simulink model "LIVA_AUV_SIMULATOR"  (R2023b)
settings: Solver=ode4  StartTime=0.0  StopTime=100  FixedStep=0.001  RelTol=0.01  EnableMultiTasking=on
InitFcn:
  | LIVA_AUV_Simulator_init;
model workspace (MAT data in the model file):
  a = 0.0768559116543
  a1 = 5.09287831845
  b = 2.78447714902
  b1 = 0.0150573456987
  c = 0.222680447107
  c1 = 0.0244981849866
  d = 1.17025942432
  d1 = -0.121090969634
  e = 4
  e1 = -0.000744741765672
  f = 3.22045295126
  f1 = 0.147531958158
  g = 3
  g1 = 9.31921319068e-05
  h = 4
  h1 = -0.000787888183232
  i = 2.39426372075
  i1 = -0.0976897881188
  j = 3
  j1 = 7.29765081481
  k = 2
  k1 = 3.34164431501
  l = -0.0819081975806
  l1 = 4.85550524224
  m = -0.0907196254339
  m1 = 2.91684244028
  n = 1.20537954163
  n1 = 9.00648148706
  o = 1.92822193114
  o1 = 2.79427167815
  p = 1.9547800679
  p1 = 9.64465760947
  r = 2
  r1 = 9.85880905818
  s = 0.00182097897058
  s1 = 6.72892013716
values from neighbouring files (symbols this model uses):
  alfa = 1.1    [LIVA_AUV_Simulator_init.m]
  B = 114.8*pk    (= 149.24)    [LIVA_AUV_Simulator_init.m]
  Hybrid_pKd = 1.9282219311449538    (= 1.92822193114)    [LIVA_AUV_Simulator_init.m]
  Hybrid_pKi = 1.205379541632126    (= 1.20537954163)    [LIVA_AUV_Simulator_init.m]
  Hybrid_pKp = -0.090719625433908213    (= -0.0907196254339)    [LIVA_AUV_Simulator_init.m]
  Hybrid_rKd = -0.0819081975805605    (= -0.0819081975806)    [LIVA_AUV_Simulator_init.m]
  Hybrid_rKi = 2    [LIVA_AUV_Simulator_init.m]
  Hybrid_rKp = 3    [LIVA_AUV_Simulator_init.m]
  Hybrid_xalfa = 5.092878318451735    (= 5.09287831845)    [LIVA_AUV_Simulator_init.m]
  Hybrid_xbeta = 0.024498184986623803    (= 0.0244981849866)    [LIVA_AUV_Simulator_init.m]
  Hybrid_xKd = 0.22268044710682114    (= 0.222680447107)    [LIVA_AUV_Simulator_init.m]
  Hybrid_xKi = 2.7844771490230995    (= 2.78447714902)    [LIVA_AUV_Simulator_init.m]
  Hybrid_xKp = 0.076855911654313547    (= 0.0768559116543)    [LIVA_AUV_Simulator_init.m]
  Hybrid_yalfa = -0.12109096963388193    (= -0.121090969634)    [LIVA_AUV_Simulator_init.m]
  Hybrid_ybeta = 0.14753195815811565    (= 0.147531958158)    [LIVA_AUV_Simulator_init.m]
  Hybrid_yKd = 3.2204529512582094    (= 3.22045295126)    [LIVA_AUV_Simulator_init.m]
  Hybrid_yKi = 4    [LIVA_AUV_Simulator_init.m]
  Hybrid_yKp = 1.1702594243169564    (= 1.17025942432)    [LIVA_AUV_Simulator_init.m]
  Hybrid_ywKd = 0.001820978970578287    (= 0.00182097897058)    [LIVA_AUV_Simulator_init.m]
  Hybrid_ywKi = 2    [LIVA_AUV_Simulator_init.m]
  Hybrid_ywKp = 1.9547800678980167    (= 1.9547800679)    [LIVA_AUV_Simulator_init.m]
  Hybrid_zalfa = 0.000093192131906777681    (= 9.31921319068e-05)    [LIVA_AUV_Simulator_init.m]
  Hybrid_zbeta = -0.097689788118772547    (= -0.0976897881188)    [LIVA_AUV_Simulator_init.m]
  Hybrid_zKd = 2.3942637207502    (= 2.39426372075)    [LIVA_AUV_Simulator_init.m]
  Hybrid_zKi = 4    [LIVA_AUV_Simulator_init.m]
  Hybrid_zKp = 3    [LIVA_AUV_Simulator_init.m]
  iPID_pKd = 0.00013750228463629022    (= 0.000137502284636)    [LIVA_AUV_Simulator_init.m]
  iPID_pKi = 0.031254576821627369    (= 0.0312545768216)    [LIVA_AUV_Simulator_init.m]
  iPID_pKp = 0    [LIVA_AUV_Simulator_init.m]
  iPID_rKd = 2    [LIVA_AUV_Simulator_init.m]
  iPID_rKi = 9.65529148649622E-19    (= 9.6552914865e-19)    [LIVA_AUV_Simulator_init.m]
  iPID_rKp = 3    [LIVA_AUV_Simulator_init.m]
  iPID_xKd = 0    [LIVA_AUV_Simulator_init.m]
  iPID_xKi = 1.1219546659293831    (= 1.12195466593)    [LIVA_AUV_Simulator_init.m]
  iPID_xKp = 0.018002365678869262    (= 0.0180023656789)    [LIVA_AUV_Simulator_init.m]
  iPID_yKd = 3.4277809029094881E-18    (= 3.42778090291e-18)    [LIVA_AUV_Simulator_init.m]
  iPID_yKi = 0.13401348623396903    (= 0.134013486234)    [LIVA_AUV_Simulator_init.m]
  iPID_yKp = 3    [LIVA_AUV_Simulator_init.m]
  iPID_ywKd = 0.62280020767048139    (= 0.62280020767)    [LIVA_AUV_Simulator_init.m]
  iPID_ywKi = 2    [LIVA_AUV_Simulator_init.m]
  iPID_ywKp = 0.87058892280816969    (= 0.870588922808)    [LIVA_AUV_Simulator_init.m]
  iPID_zKd = 0.00075053756185264819    (= 0.000750537561853)    [LIVA_AUV_Simulator_init.m]
  iPID_zKi = 3.5484685597653076    (= 3.54846855977)    [LIVA_AUV_Simulator_init.m]
  iPID_zKp = 0.26825539985723995    (= 0.268255399857)    [LIVA_AUV_Simulator_init.m]
  Ix = 0.16*pk    (= 0.208)    [LIVA_AUV_Simulator_init.m]
  Iy = 0.16*pk    (= 0.208)    [LIVA_AUV_Simulator_init.m]
  Iz = 0.16*pk    (= 0.208)    [LIVA_AUV_Simulator_init.m]
  Kc = 20*eye(6)    [LIVA_AUV_Simulator_init.m]
  Kp = 11.7*pk    (= 15.21)    [LIVA_AUV_Simulator_init.m]
  Kpdot = 0*pk    (= 0)    [LIVA_AUV_Simulator_init.m]
  Kpp = 1.55*pk    (= 2.015)    [LIVA_AUV_Simulator_init.m]
  Mq = 15*pk    (= 19.5)    [LIVA_AUV_Simulator_init.m]
  Mqdot = 0.0023*pk    (= 0.00299)    [LIVA_AUV_Simulator_init.m]
  Mqq = 1.55*pk    (= 2.015)    [LIVA_AUV_Simulator_init.m]
  Nr = 30*pk    (= 39)    [LIVA_AUV_Simulator_init.m]
  Nrdot = 0.0023*pk    (= 0.00299)    [LIVA_AUV_Simulator_init.m]
  Nrr = 1.55*pk    (= 2.015)    [LIVA_AUV_Simulator_init.m]
  PID_pKd = -0.04940918869876651    (= -0.0494091886988)    [LIVA_AUV_Simulator_init.m]
  PID_pKi = 2    [LIVA_AUV_Simulator_init.m]
  PID_pKp = -0.39327079611315297    (= -0.393270796113)    [LIVA_AUV_Simulator_init.m]
  PID_rKd = -0.054985573360707168    (= -0.0549855733607)    [LIVA_AUV_Simulator_init.m]
  PID_rKi = 0.001    [LIVA_AUV_Simulator_init.m]
  PID_rKp = -0.040345732248197354    (= -0.0403457322482)    [LIVA_AUV_Simulator_init.m]
  PID_xKd = 4    [LIVA_AUV_Simulator_init.m]
  PID_xKi = 4    [LIVA_AUV_Simulator_init.m]
  PID_xKp = 3    [LIVA_AUV_Simulator_init.m]
  PID_yKd = 3.1154066328676535    (= 3.11540663287)    [LIVA_AUV_Simulator_init.m]
  PID_yKi = 4    [LIVA_AUV_Simulator_init.m]
  PID_yKp = 3    [LIVA_AUV_Simulator_init.m]
  PID_ywKd = 0.89665765450717427    (= 0.896657654507)    [LIVA_AUV_Simulator_init.m]
  PID_ywKi = -0.006253695766722793    (= -0.00625369576672)    [LIVA_AUV_Simulator_init.m]
  PID_ywKp = 0.98566932171151178    (= 0.985669321712)    [LIVA_AUV_Simulator_init.m]
  PID_zKd = 0.01813689620732389    (= 0.0181368962073)    [LIVA_AUV_Simulator_init.m]
  PID_zKi = 4    [LIVA_AUV_Simulator_init.m]
  PID_zKp = 3    [LIVA_AUV_Simulator_init.m]
  Tmax = 40    [LIVA_AUV_Simulator_init.m]
  Ts_controller = 0.001    [LIVA_AUV_Simulator_init.m]
  twodof_palfa = 0.25    [LIVA_AUV_Simulator_init.m]
  twodof_pbeta = 0.12    [LIVA_AUV_Simulator_init.m]
  twodof_pKd = 0.095424714936744218    (= 0.0954247149367)    [LIVA_AUV_Simulator_init.m]
  twodof_pKi = 0.13825854798036114    (= 0.13825854798)    [LIVA_AUV_Simulator_init.m]
  twodof_pKp = 0.11369893762575015    (= 0.113698937626)    [LIVA_AUV_Simulator_init.m]
  twodof_ralfa = 0.19999999999999798    (= 0.2)    [LIVA_AUV_Simulator_init.m]
  twodof_rbeta = 0.20000000000000065    (= 0.2)    [LIVA_AUV_Simulator_init.m]
  twodof_rKd = 0.53578437965746184    (= 0.535784379657)    [LIVA_AUV_Simulator_init.m]
  twodof_rKi = 1.1506401605012322    (= 1.1506401605)    [LIVA_AUV_Simulator_init.m]
  twodof_rKp = 2.9999790377213507    (= 2.99997903772)    [LIVA_AUV_Simulator_init.m]
  twodof_xalfa = 0.30234710594262    (= 0.302347105943)    [LIVA_AUV_Simulator_init.m]
  twodof_xbeta = 1.7366690704427536    (= 1.73666907044)    [LIVA_AUV_Simulator_init.m]
  twodof_xKd = 0.97271920084965735    (= 0.97271920085)    [LIVA_AUV_Simulator_init.m]
  twodof_xKi = 3.9943078181304963    (= 3.99430781813)    [LIVA_AUV_Simulator_init.m]
  twodof_xKp = 0.28411216909151349    (= 0.284112169092)    [LIVA_AUV_Simulator_init.m]
  twodof_yalfa = 0.10435250246875363    (= 0.104352502469)    [LIVA_AUV_Simulator_init.m]
  twodof_ybeta = 0.005650227565256156    (= 0.00565022756526)    [LIVA_AUV_Simulator_init.m]
  twodof_yKd = 0.18997113533365648    (= 0.189971135334)    [LIVA_AUV_Simulator_init.m]
  twodof_yKi = 3.9999790377213498    (= 3.99997903772)    [LIVA_AUV_Simulator_init.m]
  twodof_yKp = 0.063666271676642031    (= 0.0636662716766)    [LIVA_AUV_Simulator_init.m]
  twodof_ywalfa = -4.2798991350061177    (= -4.27989913501)    [LIVA_AUV_Simulator_init.m]
  twodof_ywbeta = 0.35373480857737255    (= 0.353734808577)    [LIVA_AUV_Simulator_init.m]
  twodof_ywKd = 1.0659867557210738    (= 1.06598675572)    [LIVA_AUV_Simulator_init.m]
  twodof_ywKi = 0.00008440390384513819    (= 8.44039038451e-05)    [LIVA_AUV_Simulator_init.m]
  twodof_ywKp = 0.28527888951964514    (= 0.28527888952)    [LIVA_AUV_Simulator_init.m]
  twodof_zalfa = 0.00008034865340691478    (= 8.03486534069e-05)    [LIVA_AUV_Simulator_init.m]
  twodof_zbeta = 0.32801506093302246    (= 0.328015060933)    [LIVA_AUV_Simulator_init.m]
  twodof_zKd = 2.2289396936947683    (= 2.22893969369)    [LIVA_AUV_Simulator_init.m]
  twodof_zKi = 3.8840765857077431    (= 3.88407658571)    [LIVA_AUV_Simulator_init.m]
  twodof_zKp = 2.9999790377213507    (= 2.99997903772)    [LIVA_AUV_Simulator_init.m]
  W = 112.8*pk    (= 146.64)    [LIVA_AUV_Simulator_init.m]
  xb = 0    [LIVA_AUV_Simulator_init.m]
  xg = 0    [LIVA_AUV_Simulator_init.m]
  Xu = 26*pk    (= 33.8)    [LIVA_AUV_Simulator_init.m]
  Xudot = 10.6505*pk    (= 13.84565)    [LIVA_AUV_Simulator_init.m]
  Xuu = 18.18*pk    (= 23.634)    [LIVA_AUV_Simulator_init.m]
  yb = 0    [LIVA_AUV_Simulator_init.m]
  yg = 0    [LIVA_AUV_Simulator_init.m]
  Yv = 30*pk    (= 39)    [LIVA_AUV_Simulator_init.m]
  Yvdot = 11.9247*pk    (= 15.50211)    [LIVA_AUV_Simulator_init.m]
  Yvv = 21.66*pk    (= 28.158)    [LIVA_AUV_Simulator_init.m]
  zb = 0    [LIVA_AUV_Simulator_init.m]
  zg = 0.02    [LIVA_AUV_Simulator_init.m]
  ... (+3 more)
undefined symbols (not defined in the file or in its folder): DiscIntNeverNeededParam, gray, sigbuilder_block
libraries: slpidlib x29, eeGeneralControl x19, pid_lib x6, simulink x4, sim3dlib x4
(part 1 of 6)
settings Model: Creator=meteh  LastModifiedBy=Mete
settings SolverCC: AlgebraicLoopSolver=LineSearch  AutoInsertRateTranBlk=on  InsertRTBMode=Always
settings DataIOCC: ReturnWorkspaceOutputsName=SDOSimTest_Log
settings OptimizationCC: ReuseModelBlockBuffer=off
settings DebuggingCC: MaxConsecutiveZCsMsg=warning  IgnoredZcDiagnostic=none  UnconnectedInputMsg=warning  UnconnectedOutputMsg=warning  UnconnectedLineMsg=warning
settings ModelReferenceCC: EnableRefExpFcnMdlSchedulingChecks=on
settings SFSimCC: CustomCodeUndefinedFunction=UseInterfaceOnly
settings RTWCC: DLArmComputeVersion=19.05
settings ConfigComp: DVTestSuiteOptimization=Auto  DVDetectOutOfBounds=on

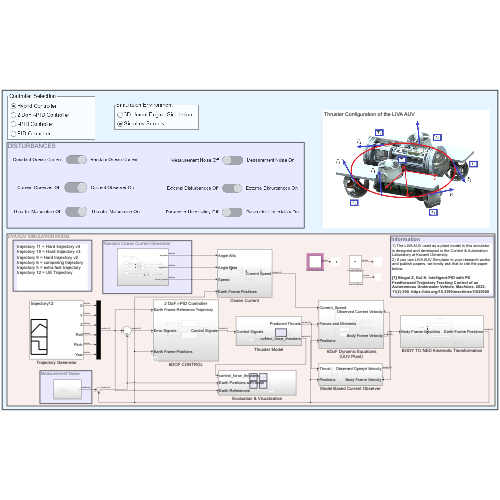
[thumbnail: Simulink's stored preview of the top-level diagram]
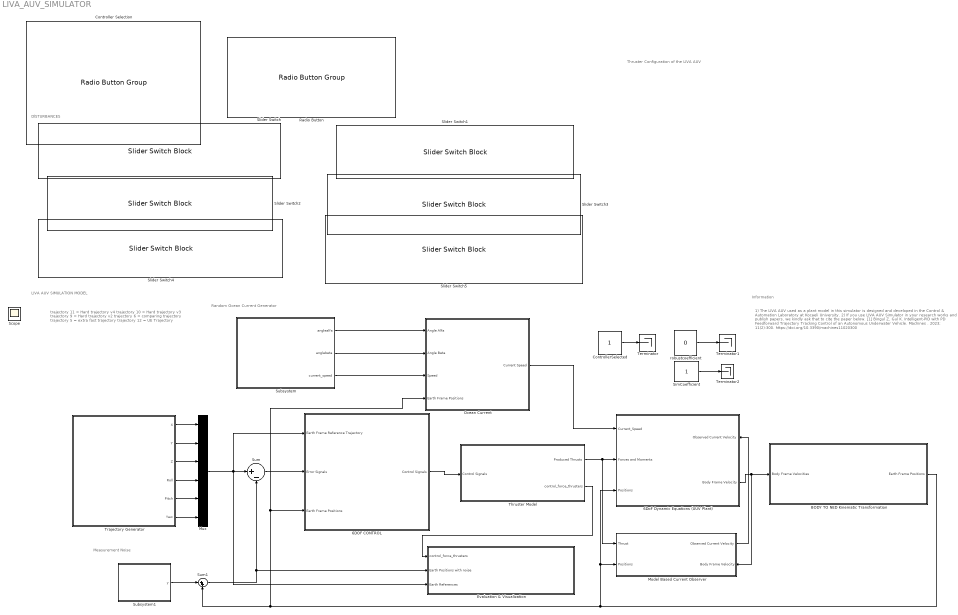
== system LIVA_AUV_SIMULATOR ==
  note: Information
  note: Thruster Configuration of the LIVA AUV
  note: trajectory 11 = Hard trajectory v4
      | trajectory 10 = Hard trajectory v3
      | trajectory 9 = Hard trajectory v2
      | trajectory 6 = comparing trajectory
      | trajectory 5 = extra fast trajectory
      | trajectory 12 = UE Trajectory
  note: LIVA AUV SIMULATION MODEL
  note: Measurement Noise
  note: Random Ocean Current Generator
  note: DİSTURBANCES
  note: 1) The LIVA AUV used as a plant model in this simulator is designed and developed in the Control & Automation Laboratory at Kocaeli University.
      | 2) If you use LIVA AUV Simulator in your research works and publish papers, we kindly ask that to cite the paper below.
      |
      | [1] Bingul Z, Gul K. Intelligent-PID with PD Feedforward Trajectory Tracking Control of an Autonomous Underwater Vehicle. Machines . 2023; 11(2):300. https://doi.org/10.3390/machines11020300
  " 6DoF Dynamic Equations (UUV Plant)" : Subsystem
      settings: PortSchema="{\"entries\":[{\"content\":{\"sides\":[{\"content\":{\"connectorIds\":[\"In1\",\"In2\",\"In3\"]},\"type\":\"ConnectorPlacement.EquallySpacedRectSide\",\"uuid\":\"68855c18-f905-4735-a86a-81e2661cb8da\"},{\"content\":{\"connectorIds\":[\"In4\",\"Out1\"],\"side\":\"RIGHT\"},\"type\":\"ConnectorPlacement.EquallySpacedRectSide\",\"uuid\":\"7717ce14-b11b-49b8-93e4-328ee3f313d1\"},{\"content\":{\"connectorIds\":[],\"side\":\"TOP\"},\"type\":\"ConnectorPlacement.EquallySpacedRectSide\",\"uuid\":\"adb132ab-47f2-49d8-8963-6702871bd2fb\"},{\"content\":{\"connectorIds\":[],\"side\":\"HIDDEN\"},\"type\":\"ConnectorPlacement.EquallySpacedRectSide\",\"uuid\":\"b80574ee-08cd-46a1-a06f-8dde445dedfc\"}]},\"type\":\"ConnectorPlacement.EquallySpacedConnector\",\"uuid\":\"92831c5d-9eed-4bec-9cab-aedecc156205\"}],\"packageUris\":[\"http://schema.mathworks.com/mf0/Connector/R2020b\"],\"version\":\"1.0\"}"
  6DOF CONTROL : Subsystem  Variant=on
  BODY TO NED Kinematic Transformation : Subsystem
  Controller Selection : RadioButtonGroup  LabelPosition=Hide  SelectedLabel=Hybrid Controller  ButtonGroupName=Controller Selection
      settings: Values={{'Hybrid Controller', '2 DoF i-PID Controller', 'i-PID Controller', 'PID Controller'}, [1 2 3 4]}
  ControllerSelected : Constant
  Evaluation & Visualization : Subsystem
  Model Based Current Observer : Subsystem
      settings: PortSchema="{\"entries\":[{\"content\":{\"sides\":[{\"content\":{\"connectorIds\":[\"In1\",\"In2\"]},\"type\":\"ConnectorPlacement.EquallySpacedRectSide\",\"uuid\":\"6a3039f9-ed18-470d-b925-a1b204af7e1a\"},{\"content\":{\"connectorIds\":[\"Out1\",\"In3\"],\"side\":\"RIGHT\"},\"type\":\"ConnectorPlacement.EquallySpacedRectSide\",\"uuid\":\"ef568844-6e92-46ac-8763-23da4c6d6096\"},{\"content\":{\"connectorIds\":[],\"side\":\"TOP\"},\"type\":\"ConnectorPlacement.EquallySpacedRectSide\",\"uuid\":\"83a932cd-173b-4c4f-a35b-7b84337aab39\"},{\"content\":{\"connectorIds\":[],\"side\":\"HIDDEN\"},\"type\":\"ConnectorPlacement.EquallySpacedRectSide\",\"uuid\":\"8f8e767e-9fc4-4dff-9aad-a0f19ac5e4b7\"}]},\"type\":\"ConnectorPlacement.EquallySpacedConnector\",\"uuid\":\"a868378d-5701-41b1-aec4-6d923424f916\"}],\"packageUris\":[\"http://schema.mathworks.com/mf0/Connector/R2020b\"],\"version\":\"1.0\"}"
  Mux : Mux  Inputs=6
  Ocean Current : Subsystem
  Radio Button : RadioButtonGroup  LabelPosition=Hide  SelectedLabel=Simulink Scopes  ButtonGroupName=Simulation Environment
      settings: Values={{'3D Unreal Engine Simulation', 'Simulink Scopes'}, [0 1]}
  SimCoefficient : Constant
  Slider Switch{,1..5} (6 alike) : SliderSwitchBlock  LabelPosition=Hide
  Subsystem : Subsystem
  Subsystem1 : Subsystem
  Sum : Sum  Inputs=|+-
  Sum1 : Sum  Inputs=|++
  Terminator : Terminator
  Terminator1 : Terminator
  Terminator2 : Terminator
  Thruster Model : Subsystem
  Trajectory Generator : Subsystem  Tag=STV Subsys  LoadFcn=sigbuilder_block('load');  StartFcn=sigbuilder_block('start');  StopFcn=sigbuilder_block('stop');  ClipboardFcn=sigbuilder_block('clipboard');  mask(Sigbuilder block){tuvar=[0:10]}
      mask help: Simulink:masks:SigbuilderBlock_MD
      mask init:
      | if ~strcmp(get_param(bdroot(gcbh),'SimulationStatus'),'stopped') tuvar = sigbuilder_block('maskInit'); end
      settings: CopyFcn=sigbuilder_block('copy');  DeleteFcn=sigbuilder_block('delete');  ModelCloseFcn=sigbuilder_block('modelClose');  PreSaveFcn=sigbuilder_block('preSave');  PauseFcn=sigbuilder_block('pause');  ContinueFcn=sigbuilder_block('continue');  NameChangeFcn=sigbuilder_block('namechange');  OpenFcn=sigbuilder_block('open',[585.75 67.5 848.25 518.25 ]);  CloseFcn=sigbuilder_block('close');
      mask Display: plot(0, 0, 100, 100,[2, 2, 32, 32, 2], [68, 8, 8, 68, 68],[32, 2], [38, 38], [32, 19, 2],[53, 60, 44], [32, 17, 17, 2],[16, 16, 31, 31]);txt = getActiveGroup(gcbh);text(2, 100, txt,'verticalAlignment', 'top');
  robustcoefficient : Constant  Value=0
  Scope : Scope
  wires:
  Mux/1 -> 6DOF CONTROL/1(Earth Frame Reference Trajectory), Evaluation & Visualization/3(Earth References), Sum/1
  6DOF CONTROL/1(Control Signals) -> Thruster Model/1(Control Signals)
  Trajectory Generator/2(Y) -> Mux/2
  Trajectory Generator/3(Z) -> Mux/3
  Trajectory Generator/5(Pitch) -> Mux/5
  Trajectory Generator/4(Roll) -> Mux/4
  Trajectory Generator/6(Yaw) -> Mux/6
  " 6DoF Dynamic Equations (UUV Plant)"/1(Body Frame Velocity) -> Model Based Current Observer/3(Body Frame Velocity), BODY TO NED Kinematic Transformation/1(Body Frame Velocities)
  Thruster Model/1(Produced Thrusts) -> Model Based Current Observer/1("Thrust "), " 6DoF Dynamic Equations (UUV Plant)"/2("Forces and Moments  ")
  Ocean Current/1(Current Speed) -> " 6DoF Dynamic Equations (UUV Plant)"/1(Current_Speed)
  Subsystem1/1(y) -> Sum1/1
  Sum1/1 -> Sum/2, Evaluation & Visualization/2(Earth Positions with noise)
  BODY TO NED Kinematic Transformation/1(Earth Frame Positions) -> Model Based Current Observer/2("Positions "), " 6DoF Dynamic Equations (UUV Plant)"/3("Positions "), Ocean Current/4(Earth Frame Positions), 6DOF CONTROL/3(Earth Frame Positions), Sum1/2
  Thruster Model/2(control_force_thrusters) -> Evaluation & Visualization/1(control_force_thrusters)
  Model Based Current Observer/1(Observed Current Velocity) -> " 6DoF Dynamic Equations (UUV Plant)"/4(Observed Current Velocity)
  Trajectory Generator/1(X) -> Mux/1
  Sum/1 -> 6DOF CONTROL/2(Error Signals)
  Subsystem/1(anglealfa) -> Ocean Current/1(Angle Alfa)
  Subsystem/2(anglebeta) -> Ocean Current/2(Angle Beta)
  Subsystem/3(current_speed) -> Ocean Current/3(Speed)
  ControllerSelected/1 -> Terminator/1
  robustcoefficient/1 -> Terminator1/1
  SimCoefficient/1 -> Terminator2/1

== system LIVA_AUV_SIMULATOR/ 6DoF Dynamic Equations (UUV Plant) ==
  Current_Speed : Inport
  "Forces and Moments  " : Inport  Port=2
  "Positions " : Inport  Port=3
  Observed Current Velocity : Inport  Port=4
  " A Matrix" : Subsystem
  "Centripetal and Coriolis Matrices " : Subsystem
  Discrete-Time Integrator : DiscreteIntegrator  SampleTime=-1  StateName=x  ICPrevOutput=DiscIntNeverNeededParam  ICPrevScaledInput=DiscIntNeverNeededParam
  "Hydrodynamic Damping Matrices " : Subsystem
  Inverse Mass Matrix : Subsystem
  Restoring Forces Matrix : Subsystem
  Scope : Scope  NumInputPorts=2
  Sum : Sum  Inputs=|+-+
  Sum1 : Sum  Inputs=+---+  InputSameDT=on  SaturateOnIntegerOverflow=on  OutDataTypeStr=Inherit: Same as first input
  Body Frame Velocity : Outport  VectorParamsAs1DForOutWhenUnconnected=off
  wires:
  Restoring Forces Matrix/1(Gravitational Force) -> Sum1/2
  "Hydrodynamic Damping Matrices "/1(Damping Force) -> Sum1/3
  "Positions "/1 -> Restoring Forces Matrix/1(positions)
  Sum1/1 -> Inverse Mass Matrix/1(Thrust force)
  "Forces and Moments  "/1 -> Sum1/1
  "Centripetal and Coriolis Matrices "/1(Coriolis Force) -> Sum1/4
  Observed Current Velocity/1 -> Sum/3, Scope/2
  Sum/1 -> "Hydrodynamic Damping Matrices "/1(Velocity), "Centripetal and Coriolis Matrices "/2(Velocity_with_current)
  Inverse Mass Matrix/1(Acceleration) -> Discrete-Time Integrator/1
  Current_Speed/1 -> Scope/1, " A Matrix"/1(currentvel), Sum/2
  Discrete-Time Integrator/1 -> Body Frame Velocity/1, Sum/1, "Centripetal and Coriolis Matrices "/1(Velocity_no_current)
  " A Matrix"/1(Ac) -> Sum1/5

== system LIVA_AUV_SIMULATOR/6DOF CONTROL ==
  Earth Frame Reference Trajectory : Inport
  Error Signals : Inport  Port=2
  Earth Frame Positions : Inport  Port=3
  2 DoF i-PID Controller : Subsystem  VariantControl=(get_param([bdroot '/ControllerSelected'], 'Value') == '2')
  Hybrid i-PID Controller : Subsystem  VariantControl=(get_param([bdroot '/ControllerSelected'], 'Value') == '1')
  "PID Controller " : Subsystem  VariantControl=(get_param([bdroot '/ControllerSelected'], 'Value') == '4')
  i-PID Controler : Subsystem  VariantControl=(get_param([bdroot '/ControllerSelected'], 'Value') == '3')
  Control Signals : Outport

== system LIVA_AUV_SIMULATOR/BODY TO NED Kinematic Transformation ==
  note: Body Frame Positions
  note: u[1 2 3 4 5 6]
  note: u[7 8 9 10 11 12]
  note: NED(v) = J(n)*BODY(v)
  Body Frame Velocities : Inport
  Fcn10 : Fcn  Expr=cos(u[10])*u[5]-sin(u[10])*u[6]
  Fcn11 : Fcn  Expr=(sin(u[10])/cos(u[11]))*u[5]+(cos(u[10])/cos(u[11]))*u[6]
  Fcn6 : Fcn  Expr=(cos(u[12])*cos(u[11])*u[1]-sin(u[12])*cos(u[10])*u[2]+cos(u[12])*sin(u[11])*sin(u[10])*u[2]+sin(u[12])*sin(u[10])*u[3]+cos(u[12])*cos(u[10])*sin(u[11])*u[3])
  Fcn7 : Fcn  Expr=sin(u[12])*cos(u[11])*u[1]+cos(u[12])*cos(u[10])*u[2]+sin(u[10])*sin(u[11])*sin(u[12])*u[2]-cos(u[12])*sin(u[10])*u[3]+sin(u[11])*sin(u[12])*cos(u[11])*u[3]
  Fcn8 : Fcn  Expr=-sin(u[11])*u[1]+cos(u[11])*sin(u[10])*u[2]+cos(u[11])*cos(u[10])*u[3]
  Fcn9 : Fcn  Expr=u[4]+sin(u[10])*tan(u[11])*u[5]+cos(u[10])*tan(u[11])*u[6]
  Integrator Block : Subsystem
  Mux2 : Mux  Inputs=2
  Mux3 : Mux  Inputs=6
  To Workspace : ToWorkspace  VariableName=simout25  SampleTime=-1
  Earth Frame Positions : Outport
  wires:
  Fcn11/1 -> Mux3/6
  Fcn10/1 -> Mux3/5
  Fcn9/1 -> Mux3/4
  Mux3/1 -> To Workspace/1, Integrator Block/1(Velocities)
  Fcn8/1 -> Mux3/3
  Fcn6/1 -> Mux3/1
  Integrator Block/1(Positions) -> Mux2/2, Earth Frame Positions/1
  Fcn7/1 -> Mux3/2
  Mux2/1 -> Fcn11/1, Fcn10/1, Fcn9/1, Fcn8/1, Fcn7/1, Fcn6/1
  Body Frame Velocities/1 -> Mux2/1

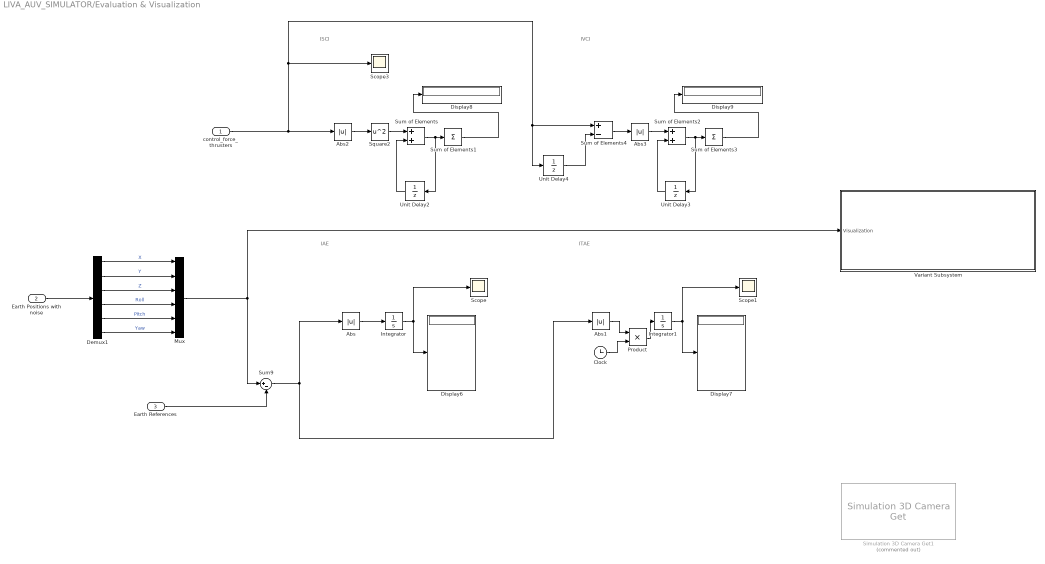
== system LIVA_AUV_SIMULATOR/Evaluation & Visualization ==
  note: ISCI
  note: IAE
  note: ITAE
  note: IVCI
  control_force_thrusters : Inport
  Earth Positions with noise : Inport  Port=2
  Earth References : Inport  Port=3
  Abs{,1..3} (4 alike) : Abs  SaturateOnIntegerOverflow=off
  Clock : Clock
  Demux1 : Demux  Outputs=6
  Display{6..9} (4 alike) : Display
  Integrator : Integrator
  Integrator1 : Integrator
  Mux : Mux  Inputs=6
  Product : Product
  Scope : Scope
  Scope1 : Scope
  Scope3 : Scope
  Simulation 3D Camera Get1 : sim3dlib/Simulation 3D Camera Get  Priority=1  Commented=on  sensorTag=Sim3dSensor2  sensorId=2  sensorName=Sim3dSensor2  vehTagList={'Scene Origin'}  vehTag=Scene Origin  mountLoc=Origin  offsetFlag=on  tmountOffset=[6.5, 13.5, 12]  rmountOffset=[0, 25, 225]  HorizontalResolution=1280  VerticalResolution=720  HorizontalFOV=120  SampleTime=-1  mountPoint=[6.5 -13.5 12]  mountOrientation=[0 -25 -225]  aMode=2  ID=2
      settings: LibrarySourceBlock=vehdynlibsim3dcore/Simulation 3D Camera Get
  Square2 : Math  Operator=square
  Sum of Elements : Sum
  Sum of Elements1 : Sum  Inputs=+
  Sum of Elements2 : Sum
  Sum of Elements3 : Sum  Inputs=+
  Sum of Elements4 : Sum  Inputs=+-
  Sum9 : Sum  Inputs=|+-
  Unit Delay2 : UnitDelay  SampleTime=-1  HasFrameUpgradeWarning=on
  Unit Delay3 : UnitDelay  SampleTime=-1  HasFrameUpgradeWarning=on
  Unit Delay4 : UnitDelay  SampleTime=-1  HasFrameUpgradeWarning=on
  Variant Subsystem : Subsystem  Variant=on
  wires:
  Earth References/1 -> Sum9/2
  Integrator/1 -> Scope/1, Display6/1
  Abs/1 -> Integrator/1
  Product/1 -> Integrator1/1
  Integrator1/1 -> Scope1/1, Display7/1
  Abs1/1 -> Product/1
  Clock/1 -> Product/2
  Sum9/1 -> Abs/1, Abs1/1
  Sum of Elements/1 -> Sum of Elements1/1, Unit Delay2/1
  Unit Delay2/1 -> Sum of Elements/2
  Abs2/1 -> Square2/1
  Square2/1 -> Sum of Elements/1
  Sum of Elements1/1 -> Display8/1
  Abs3/1 -> Sum of Elements2/1
  Sum of Elements3/1 -> Display9/1
  control_force_thrusters/1 -> Abs2/1, Scope3/1, Sum of Elements4/1, Unit Delay4/1
  Unit Delay3/1 -> Sum of Elements2/2
  Sum of Elements2/1 -> Sum of Elements3/1, Unit Delay3/1
  Unit Delay4/1 -> Sum of Elements4/2
  Sum of Elements4/1 -> Abs3/1
  Mux/1 -> Sum9/1, Variant Subsystem/1(Visualization)
  Demux1/1 -> Mux/1  "X"
  Demux1/2 -> Mux/2  "Y"
  Demux1/3 -> Mux/3  "Z"
  Demux1/4 -> Mux/4  "Roll"
  Demux1/5 -> Mux/5  "Pitch"
  Demux1/6 -> Mux/6  "Yaw"
  Earth Positions with noise/1 -> Demux1/1

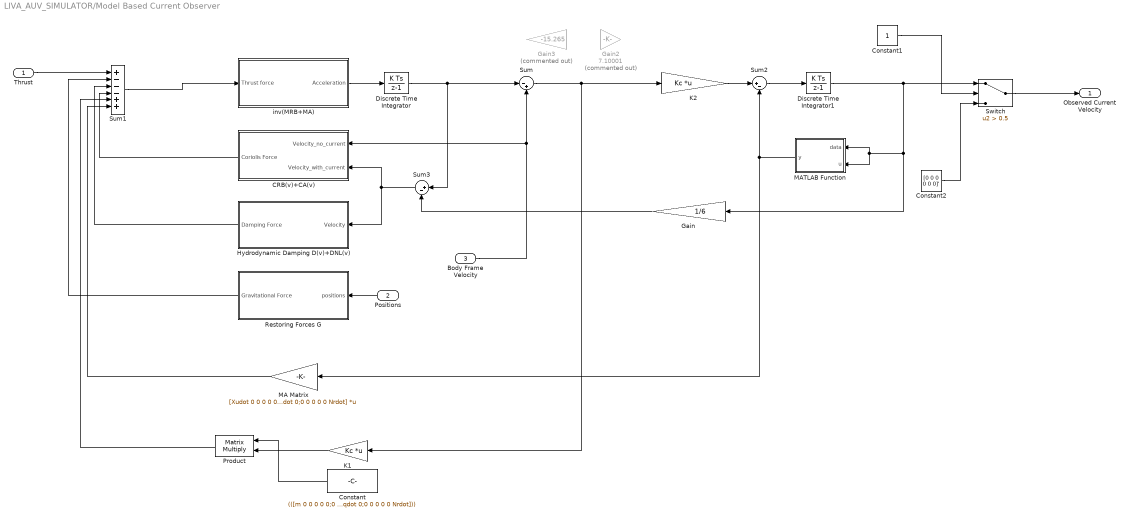
== system LIVA_AUV_SIMULATOR/Model Based Current Observer ==
  "Thrust " : Inport
  "Positions " : Inport  Port=2
  Body Frame Velocity : Inport  Port=3
  CRB(v)+CA(v) : Subsystem
  Constant : Constant  Value=(([m 0 0 0 0 0;0 m 0 0 0 0;0 0 m 0 0 0;0 0 0 Ix 0 0;0 0 0 0 Iy 0;0 0 0 0 0 Iz]+[Xudot 0 0 0 0 0;0 Yvdot 0 0 0 0;0 0 Zwdot 0 0 0;0 0 0 Kpdot 0 0;0 0 0 0 Mqdot 0;0 0 0 0 0 Nrdot]))
  Constant1 : Constant
  Constant2 : Constant  Value=[0 0 0 0 0 0]'
  Discrete Time Integrator : DiscreteIntegrator  SampleTime=-1  ICPrevOutput=DiscIntNeverNeededParam  ICPrevScaledInput=DiscIntNeverNeededParam
  Discrete Time Integrator1 : DiscreteIntegrator  SampleTime=-1  ICPrevOutput=DiscIntNeverNeededParam  ICPrevScaledInput=DiscIntNeverNeededParam
  Gain : Gain  Gain=1/6
  Gain2 : Gain  Commented=on  Gain=7.10001
  Gain3 : Gain  Commented=on  Gain=-15.265
  Hydrodynamic Damping D(v)+DNL(v) : Subsystem
  K1 : Gain  Gain=Kc  Multiplication=Matrix(K*u)
  K2 : Gain  Gain=Kc  Multiplication=Matrix(K*u)
  MA Matrix : Gain  Gain=[Xudot 0 0 0 0 0;0 Yvdot 0 0 0 0;0 0 Zwdot 0 0 0;0 0 0 Kpdot 0 0;0 0 0 0 Mqdot 0;0 0 0 0 0 Nrdot]  Multiplication=Matrix(K*u)  OutDataTypeStr=Inherit: Same as input  ParamDataTypeStr=Inherit: Same as input
  MATLAB Function : MATLAB Function  TreatAsAtomicUnit=on
  Product : Product  Multiplication=Matrix(*)
  "Restoring Forces G " : Subsystem
  Sum : Sum  Inputs=|-+
  Sum1 : Sum  Inputs=+---++  InputSameDT=on  SaturateOnIntegerOverflow=on  OutDataTypeStr=Inherit: Same as first input
  Sum2 : Sum  Inputs=|+-
  Sum3 : Sum  Inputs=|+-
  Switch : Switch  Criteria=u2 > Threshold  Threshold=0.5  SaturateOnIntegerOverflow=off  InputSameDT=off
  inv(MRB+MA) : Subsystem
  Observed Current Velocity : Outport  VectorParamsAs1DForOutWhenUnconnected=off
  wires:
  "Restoring Forces G "/1(Gravitational Force) -> Sum1/2
  Hydrodynamic Damping D(v)+DNL(v)/1(Damping Force) -> Sum1/3
  inv(MRB+MA)/1(Acceleration) -> Discrete Time Integrator/1
  "Positions "/1 -> "Restoring Forces G "/1(positions)
  Sum1/1 -> inv(MRB+MA)/1(Thrust force)
  "Thrust "/1 -> Sum1/1
  CRB(v)+CA(v)/1(Coriolis Force) -> Sum1/4
  Discrete Time Integrator/1 -> Sum3/1, Sum/1
  Product/1 -> Sum1/5
  K2/1 -> Sum2/1
  Sum3/1 -> Hydrodynamic Damping D(v)+DNL(v)/1(Velocity), CRB(v)+CA(v)/2(Velocity_with_current)
  Sum2/1 -> Discrete Time Integrator1/1
  Discrete Time Integrator1/1 -> MATLAB Function/1(data), MATLAB Function/2(u), Gain/1, Switch/1
  Body Frame Velocity/1 -> Sum/2, CRB(v)+CA(v)/1(Velocity_no_current)
  K1/1 -> Product/2
  Constant/1 -> Product/1
  Sum/1 -> K2/1, K1/1
  MATLAB Function/1(y) -> MA Matrix/1, Sum2/2
  Gain/1 -> Sum3/2
  MA Matrix/1 -> Sum1/6
  Switch/1 -> Observed Current Velocity/1
  Constant1/1 -> Switch/2
  Constant2/1 -> Switch/3

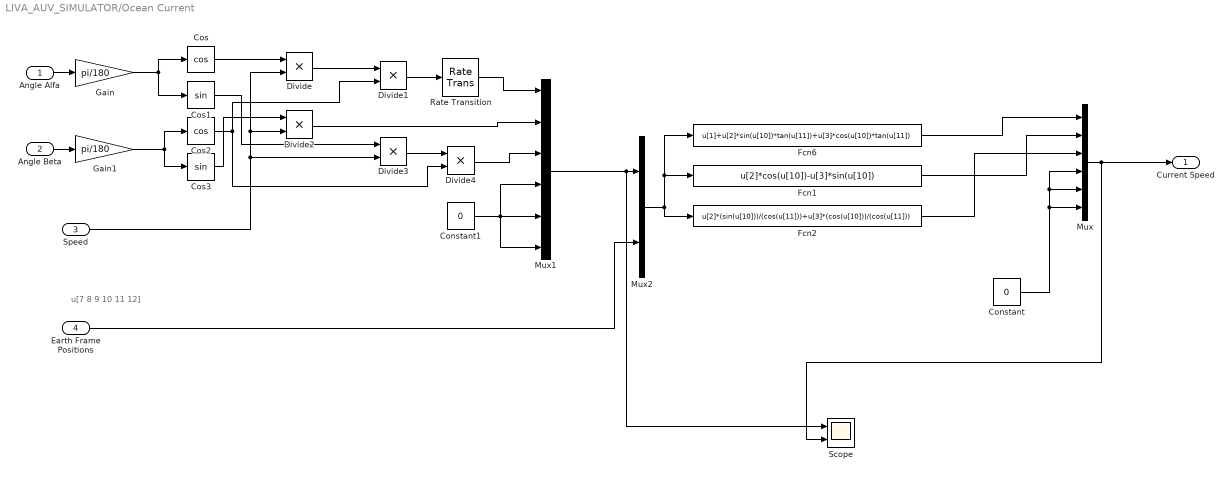
== system LIVA_AUV_SIMULATOR/Ocean Current ==
  note: u[7 8 9 10 11 12]
  Angle Alfa : Inport
  Angle Beta : Inport  Port=2
  Speed : Inport  Port=3
  Earth Frame Positions : Inport  Port=4
  Constant : Constant  Value=0
  Constant1 : Constant  Value=0
  Cos : Trigonometry  Operator=cos
  Cos1 : Trigonometry
  Cos2 : Trigonometry  Operator=cos
  Cos3 : Trigonometry
  Divide{,1..4} (5 alike) : Product  Inputs=**
  Fcn1 : Fcn  Expr=u[2]*cos(u[10])-u[3]*sin(u[10])
  Fcn2 : Fcn  Expr=u[2]*(sin(u[10]))/(cos(u[11]))+u[3]*(cos(u[10]))/(cos(u[11]))
  Fcn6 : Fcn  Expr=u[1]+u[2]*sin(u[10])*tan(u[11])+u[3]*cos(u[10])*tan(u[11])
  Gain : Gain  Gain=pi/180
  Gain1 : Gain  Gain=pi/180
  Mux : Mux  Inputs=6
  Mux1 : Mux  Inputs=6
  Mux2 : Mux  Inputs=2
  Rate Transition : RateTransition
  Scope : Scope  NumInputPorts=2
  Current Speed : Outport
  wires:
  Angle Alfa/1 -> Gain/1
  Gain/1 -> Cos/1, Cos1/1
  Mux/1 -> Scope/2, Current Speed/1
  Constant/1 -> Mux/6, Mux/5, Mux/4
  Angle Beta/1 -> Gain1/1
  Gain1/1 -> Cos3/1, Cos2/1
  Cos/1 -> Divide/1
  Speed/1 -> Divide3/2, Divide2/2, Divide/2
  Cos2/1 -> Divide4/2, Divide1/2
  Divide/1 -> Divide1/1
  Divide1/1 -> Rate Transition/1
  Cos3/1 -> Divide2/1
  Divide2/1 -> Mux1/2
  Cos1/1 -> Divide3/1
  Divide3/1 -> Divide4/1
  Divide4/1 -> Mux1/3
  Constant1/1 -> Mux1/4, Mux1/6, Mux1/5
  Mux1/1 -> Scope/1, Mux2/1
  Earth Frame Positions/1 -> Mux2/2
  Mux2/1 -> Fcn1/1, Fcn6/1, Fcn2/1
  Fcn6/1 -> Mux/1
  Fcn1/1 -> Mux/2
  Fcn2/1 -> Mux/3
  Rate Transition/1 -> Mux1/1

== system LIVA_AUV_SIMULATOR/Subsystem ==
  Constant : Constant
  Constant2 : Constant  Value=45
  Random Number : RandomNumber  Mean=45  Variance=45  Seed=1  SampleTime=5
  Random Number1 : RandomNumber  Variance=0.02  Seed=0.025  SampleTime=5
  Random Number2 : RandomNumber  Mean=45  Variance=45  Seed=1  SampleTime=5
  Sum2 : Sum  Inputs=|++
  Switch : Switch  Criteria=u2 > Threshold  Threshold=0.5  SaturateOnIntegerOverflow=off  InputSameDT=off
  Switch1 : Switch  Criteria=u2 > Threshold  Threshold=0.5  SaturateOnIntegerOverflow=off  InputSameDT=off
  Switch2 : Switch  Criteria=u2 > Threshold  Threshold=0.5  SaturateOnIntegerOverflow=off  InputSameDT=off
  average current speed(m/s) : Constant  Value=0.5
  anglealfa : Outport
  anglebeta : Outport  Port=2
  current_speed : Outport  Port=3
  wires:
  Random Number1/1 -> Sum2/1
  Constant/1 -> Switch2/2, Switch1/2, Switch/2
  Constant2/1 -> Switch1/3, Switch/3
  average current speed(m/s)/1 -> Switch2/3, Sum2/2
  Sum2/1 -> Switch2/1
  Switch2/1 -> current_speed/1
  Switch/1 -> anglealfa/1
  Switch1/1 -> anglebeta/1
  Random Number/1 -> Switch/1
  Random Number2/1 -> Switch1/1

== system LIVA_AUV_SIMULATOR/Subsystem1 ==
  note: Current noises = 10cm position + 2.2 degree orientation noise
  note: Limits = 25cm poisition noise + 9 degree orientation noise
  note: 1 deg = 0.0174532925 rad
  Band-Limited White Noise1 : simulink/Sources/Band-Limited White Noise  Cov=[0.0000001]  Ts=0.001  seed=[23341]
  Band-Limited White Noise2 : simulink/Sources/Band-Limited White Noise  Cov=[0.0000008]  Ts=0.001  seed=[23341]
  Constant : Constant  Value=[0 0 0 0 0 0]'
  Constant1 : Constant  Value=0
  Mux1 : Mux  Inputs=6
  Switch : Switch  Criteria=u2 > Threshold  SaturateOnIntegerOverflow=off  InputSameDT=off
  y : Outport
  wires:
  Band-Limited White Noise1/1 -> Mux1/6, Mux1/4, Mux1/5
  Band-Limited White Noise2/1 -> Mux1/3, Mux1/1, Mux1/2
  Switch/1 -> y/1
  Mux1/1 -> Switch/1
  Constant/1 -> Switch/3
  Constant1/1 -> Switch/2

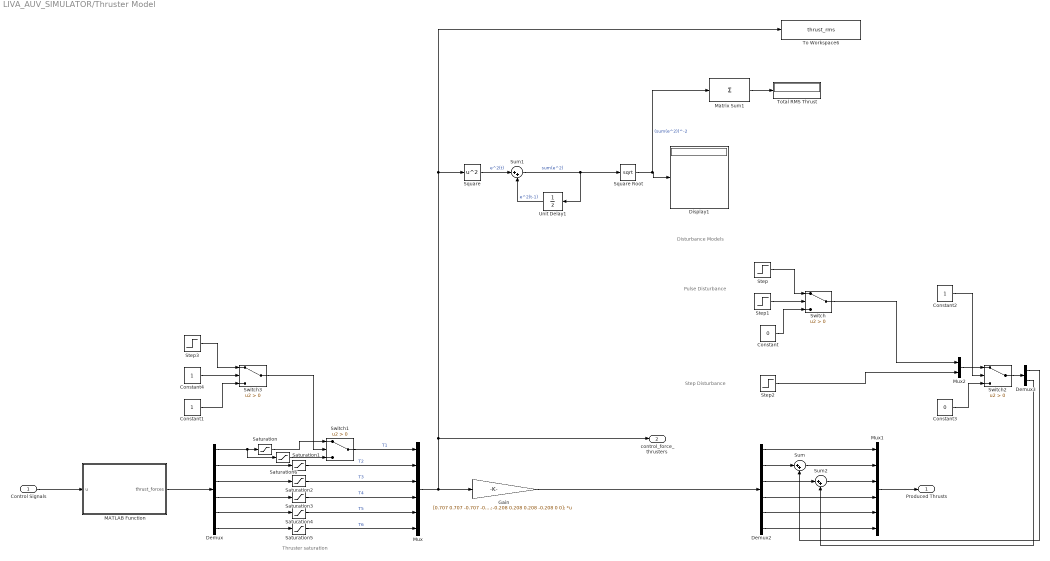
== system LIVA_AUV_SIMULATOR/Thruster Model ==
  note: Step Disturbance
  note: Pulse Disturbance
  note: Disturbance Models
  note: Thruster saturation
  Control Signals : Inport
  Constant : Constant  Value=0
  Constant1 : Constant
  Constant2 : Constant
  Constant3 : Constant  Value=0
  Constant4 : Constant
  Demux : Demux  Outputs=6
  Demux2 : Demux  Outputs=6
  Demux3 : Demux  Outputs=2
  Display1 : Display
  Gain : Gain  Gain=[0.707 0.707 -0.707 -0.707 0 0;-0.707 0.707 -0.707 0.707 0 0;0 0 0 0 1 1;-0.054 0.054 -0.054 0.054 0.127 -0.127;0.054 0.054 -0.054 -0.054 0 0;-0.208 0.208 0.208 -0.208 0 0];  Multiplication=Matrix(K*u)
  MATLAB Function : MATLAB Function  TreatAsAtomicUnit=on
  Matrix Sum1 : Sum  Inputs=+
  Mux : Mux  Inputs=6
  Mux1 : Mux  Inputs=6
  Mux2 : Mux  Inputs=2
  Saturation{,1..5} (6 alike) : Saturate  UpperLimit=Tmax  LowerLimit=-Tmax
  Saturation6 : Saturate  UpperLimit=Tmax/4  LowerLimit=-Tmax/4
  Square : Math  Operator=square
  Square Root : Sqrt
  Step : Step  Time=60  Before=-40  After=0  SampleTime=0
  Step1 : Step  Time=50  SampleTime=0
  Step2 : Step  Time=75  After=40  SampleTime=0
  Step3 : Step  Time=30  Before=1  After=0  SampleTime=0
  Sum : Sum  Inputs=|++
  Sum1 : Sum  Inputs=|++
  Sum2 : Sum  Inputs=|++
  Switch{,1..3} (4 alike) : Switch  Criteria=u2 > Threshold  SaturateOnIntegerOverflow=off  InputSameDT=off
  To Workspace6 : ToWorkspace  VariableName=thrust_rms  SampleTime=-1
  Total RMS Thrust : Display
  Unit Delay1 : UnitDelay  SampleTime=-1  HasFrameUpgradeWarning=on
  Produced Thrusts : Outport
  control_force_thrusters : Outport  Port=2
  wires:
  Control Signals/1 -> MATLAB Function/1(u)
  Demux/4 -> Saturation3/1
  Saturation3/1 -> Mux/4  "T4"
  Saturation2/1 -> Mux/3  "T3"
  Demux/6 -> Saturation5/1
  Saturation/1 -> Switch1/1
  Saturation1/1 -> Mux/2  "T2"
  Demux/2 -> Saturation1/1
  Demux/5 -> Saturation4/1
  Demux/3 -> Saturation2/1
  Mux/1 -> To Workspace6/1, Square/1, control_force_thrusters/1, Gain/1
  Saturation4/1 -> Mux/5  "T5"
  Demux2/3 -> Sum2/1
  Demux2/2 -> Sum/1
  Mux1/1 -> Produced Thrusts/1
  Step/1 -> Switch/1
  Constant/1 -> Switch/3
  Gain/1 -> Demux2/1
  Saturation5/1 -> Mux/6  "T6"
  Saturation6/1 -> Switch1/3
  Switch1/1 -> Mux/1  "T1"
  Demux/1 -> Saturation/1, Saturation6/1
  Unit Delay1/1 -> Sum1/2  "e^2(t-1)"
  Sum1/1 -> Square Root/1, Unit Delay1/1  "sum(e^2)"
  Square Root/1 -> Matrix Sum1/1, Display1/1  "(sum(e^2))^-2"
  Matrix Sum1/1 -> Total RMS Thrust/1
  Square/1 -> Sum1/1  "e^2(t)"
  Switch3/1 -> Switch1/2
  Demux2/1 -> Mux1/1
  Sum/1 -> Mux1/2
  Sum2/1 -> Mux1/3
  Demux2/4 -> Mux1/4
  Demux2/5 -> Mux1/5
  Demux2/6 -> Mux1/6
  Step1/1 -> Switch/2
  MATLAB Function/1(thrust_forces) -> Demux/1
  Switch/1 -> Mux2/1
  Step2/1 -> Mux2/2
  Demux3/1 -> Sum/2
  Demux3/2 -> Sum2/2
  Switch2/1 -> Demux3/1
  Mux2/1 -> Switch2/1
  Constant2/1 -> Switch2/2
  Constant3/1 -> Switch2/3
  Step3/1 -> Switch3/1
  Constant1/1 -> Switch3/3
  Constant4/1 -> Switch3/2

== system LIVA_AUV_SIMULATOR/Trajectory Generator ==
  Demux : Demux  Tag=STV Demux  Outputs=6
      settings: DisplayOption=none
  FromWs : FromWorkspace  Tag=STV FromWs  VariableName=tuvar
  X : Outport  Tag=STV Outport  VectorParamsAs1DForOutWhenUnconnected=off
  Y : Outport  Tag=STV Outport  Port=2  VectorParamsAs1DForOutWhenUnconnected=off
  Z : Outport  Tag=STV Outport  Port=3  VectorParamsAs1DForOutWhenUnconnected=off
  Roll : Outport  Tag=STV Outport  Port=4  VectorParamsAs1DForOutWhenUnconnected=off
  Pitch : Outport  Tag=STV Outport  Port=5  VectorParamsAs1DForOutWhenUnconnected=off
  Yaw : Outport  Tag=STV Outport  Port=6  VectorParamsAs1DForOutWhenUnconnected=off
  wires:
  Demux/6 -> Yaw/1
  Demux/5 -> Pitch/1
  Demux/4 -> Roll/1
  Demux/3 -> Z/1
  Demux/2 -> Y/1
  FromWs/1 -> Demux/1
  Demux/1 -> X/1

== system LIVA_AUV_SIMULATOR/ 6DoF Dynamic Equations (UUV Plant)/ A Matrix ==
  currentvel : Inport
  MA : Gain  Gain=[Xudot 0 0 0 0 0;0 Yvdot 0 0 0 0;0 0 Zwdot 0 0 0;0 0 0 Kpdot 0 0;0 0 0 0 Mqdot 0;0 0 0 0 0 Nrdot]  Multiplication=Matrix(K*u)  OutDataTypeStr=Inherit: Same as input  ParamDataTypeStr=Inherit: Same as input
  MATLAB Function : MATLAB Function  TreatAsAtomicUnit=on
  Ac : Outport
  wires:
  MATLAB Function/1(y) -> MA/1
  MA/1 -> Ac/1
  currentvel/1 -> MATLAB Function/1(data), MATLAB Function/2(u)

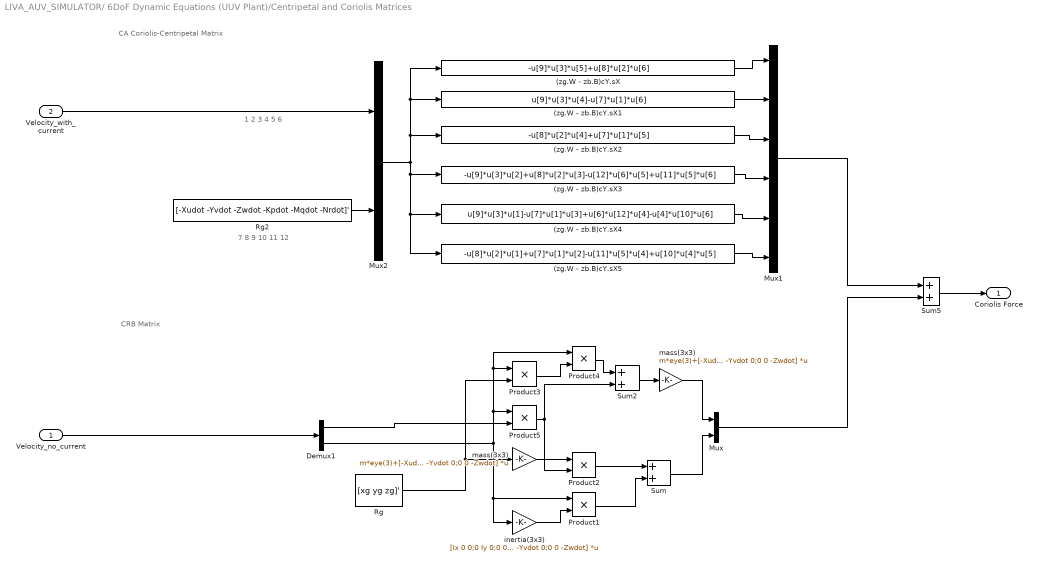
== system LIVA_AUV_SIMULATOR/ 6DoF Dynamic Equations (UUV Plant)/Centripetal and Coriolis Matrices  ==
  note: CA Coriolis-Centripetal Matrix
  note: CRB Matrix
  note: 7 8 9 10 11 12
  note: 1 2 3 4 5 6
  Velocity_no_current : Inport
  Velocity_with_current : Inport  Port=2
  (zg.W - zb.B)cY.sX : Fcn  Expr=-u[9]*u[3]*u[5]+u[8]*u[2]*u[6]
  (zg.W - zb.B)cY.sX1 : Fcn  Expr=u[9]*u[3]*u[4]-u[7]*u[1]*u[6]
  (zg.W - zb.B)cY.sX2 : Fcn  Expr=-u[8]*u[2]*u[4]+u[7]*u[1]*u[5]
  (zg.W - zb.B)cY.sX3 : Fcn  Expr=-u[9]*u[3]*u[2]+u[8]*u[2]*u[3]-u[12]*u[6]*u[5]+u[11]*u[5]*u[6]
  (zg.W - zb.B)cY.sX4 : Fcn  Expr=u[9]*u[3]*u[1]-u[7]*u[1]*u[3]+u[6]*u[12]*u[4]-u[4]*u[10]*u[6]
  (zg.W - zb.B)cY.sX5 : Fcn  Expr=-u[8]*u[2]*u[1]+u[7]*u[1]*u[2]-u[11]*u[5]*u[4]+u[10]*u[4]*u[5]
  Demux1 : Demux  Outputs=2
  Mux : Mux  Inputs=2
  Mux1 : Mux  Inputs=6
  Mux2 : Mux  Inputs=2
  Product{1..5} (5 alike) : Product  InputSameDT=on  RndMeth=Zero  SaturateOnIntegerOverflow=on  OutDataTypeStr=Inherit: Same as first input
  Rg : Constant  Value=[xg yg zg]'
  Rg2 : Constant  Value=[-Xudot -Yvdot -Zwdot -Kpdot -Mqdot -Nrdot]'
  Sum : Sum  InputSameDT=on  SaturateOnIntegerOverflow=on  OutDataTypeStr=Inherit: Same as first input
  Sum2 : Sum  InputSameDT=on  SaturateOnIntegerOverflow=on  OutDataTypeStr=Inherit: Same as first input
  Sum5 : Sum  InputSameDT=on  SaturateOnIntegerOverflow=on  OutDataTypeStr=Inherit: Same as first input
  inertia(3x3) : Gain  Gain=[Ix 0 0;0 Iy 0;0 0 Iz]*eye(3)+[-Xudot 0 0;0 -Yvdot 0;0 0 -Zwdot]  Multiplication=Matrix(K*u)  SaturateOnIntegerOverflow=on  OutDataTypeStr=Inherit: Same as input  ParamDataTypeStr=Inherit: Same as input
  "mass(3x3) " : Gain  Gain=m*eye(3)+[-Xudot 0 0;0 -Yvdot 0;0 0 -Zwdot]  Multiplication=Matrix(K*u)  SaturateOnIntegerOverflow=on  OutDataTypeStr=Inherit: Same as input  ParamDataTypeStr=Inherit: Same as input
  "mass(3x3) " : Gain  Gain=m*eye(3)+[-Xudot 0 0;0 -Yvdot 0;0 0 -Zwdot]  Multiplication=Matrix(K*u)  SaturateOnIntegerOverflow=on  OutDataTypeStr=Inherit: Same as input  ParamDataTypeStr=Inherit: Same as input
  Coriolis Force : Outport  VectorParamsAs1DForOutWhenUnconnected=off
  wires:
  (zg.W - zb.B)cY.sX2/1 -> Mux1/3
  (zg.W - zb.B)cY.sX/1 -> Mux1/1
  (zg.W - zb.B)cY.sX3/1 -> Mux1/4
  Rg2/1 -> Mux2/2
  (zg.W - zb.B)cY.sX4/1 -> Mux1/5
  (zg.W - zb.B)cY.sX1/1 -> Mux1/2
  Mux2/1 -> (zg.W - zb.B)cY.sX/1, (zg.W - zb.B)cY.sX1/1, (zg.W - zb.B)cY.sX2/1, (zg.W - zb.B)cY.sX5/1, (zg.W - zb.B)cY.sX4/1, (zg.W - zb.B)cY.sX3/1
  (zg.W - zb.B)cY.sX5/1 -> Mux1/6
  Demux1/1 -> Product5/2
  Sum/1 -> Mux/2
  "mass(3x3) "/1 -> Product2/1
  "mass(3x3) "/1 -> Mux/1
  Velocity_no_current/1 -> Demux1/1
  Product4/1 -> Sum2/1
  Demux1/2 -> Product5/1, Product3/1, Product4/1, Product1/1, inertia(3x3)/1
  Rg/1 -> Product3/2, "mass(3x3) "/1
  Sum2/1 -> "mass(3x3) "/1
  Product5/1 -> Product2/2, Sum2/2
  inertia(3x3)/1 -> Product1/2
  Product3/1 -> Product4/2
  Product1/1 -> Sum/2
  Product2/1 -> Sum/1
  Sum5/1 -> Coriolis Force/1
  Mux1/1 -> Sum5/1
  Mux/1 -> Sum5/2
  Velocity_with_current/1 -> Mux2/1

== system LIVA_AUV_SIMULATOR/ 6DoF Dynamic Equations (UUV Plant)/Hydrodynamic Damping Matrices  ==
  note: DL(v)+DNL(v)
  Velocity : Inport
  D linear : Gain  Gain=diag([Xu 0 0 0 0 0;0 Yv 0 0 0 0;0 0 Zw 0 0 0;0 0 0 Kp 0 0;0 0 0 0 Mq 0;0 0 0 0 0 Nr])  SaturateOnIntegerOverflow=on  OutDataTypeStr=Inherit: Same as input  ParamDataTypeStr=Inherit: Same as input
  D quadratic : Gain  Gain=diag([Xuu 0 0 0 0 0;0 Yvv 0 0 0 0;0 0 Zww 0 0 0;0 0 0 Kpp 0 0;0 0 0 0 Mqq 0;0 0 0 0 0 Nrr])  SaturateOnIntegerOverflow=on  OutDataTypeStr=Inherit: Same as input  ParamDataTypeStr=Inherit: Same as input
  Product : Product  InputSameDT=on  RndMeth=Zero  SaturateOnIntegerOverflow=on  OutDataTypeStr=Inherit: Same as first input
  Sum2 : Sum  InputSameDT=on  SaturateOnIntegerOverflow=on  OutDataTypeStr=Inherit: Same as first input
  |u| : Abs
  Damping Force : Outport
  wires:
  Product/1 -> Sum2/1
  |u|/1 -> D quadratic/1
  Sum2/1 -> Damping Force/1
  D linear/1 -> Sum2/2
  D quadratic/1 -> Product/2
  Velocity/1 -> D linear/1, Product/1, |u|/1

== system LIVA_AUV_SIMULATOR/ 6DoF Dynamic Equations (UUV Plant)/Inverse Mass Matrix ==
  Thrust force : Inport
  inv(MRB+MA) : Gain  Gain=inv([m 0 0 0 0 0;0 m 0 0 0 0;0 0 m 0 0 0;0 0 0 Ix 0 0;0 0 0 0 Iy 0;0 0 0 0 0 Iz]+[Xudot 0 0 0 0 0;0 Yvdot 0 0 0 0;0 0 Zwdot 0 0 0;0 0 0 Kpdot 0 0;0 0 0 0 Mqdot 0;0 0 0 0 0 Nrdot])  Multiplication=Matrix(K*u)  OutDataTypeStr=Inherit: Same as input  ParamDataTypeStr=Inherit: Same as input
  Acceleration : Outport  VectorParamsAs1DForOutWhenUnconnected=off
  wires:
  inv(MRB+MA)/1 -> Acceleration/1
  Thrust force/1 -> inv(MRB+MA)/1

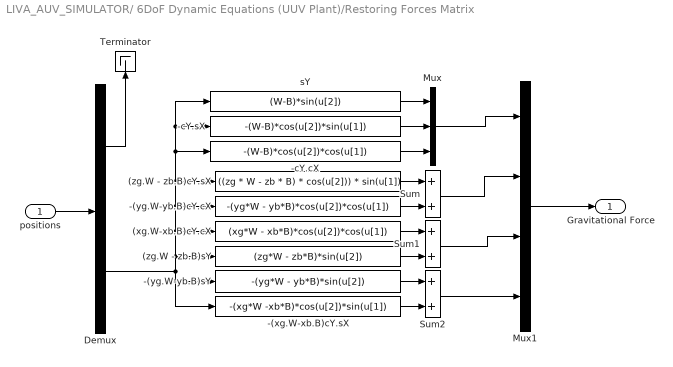
== system LIVA_AUV_SIMULATOR/ 6DoF Dynamic Equations (UUV Plant)/Restoring Forces Matrix ==
  positions : Inport
  (xg.W-xb.B)cY.cX : Fcn  Expr=(xg*W - xb*B)*cos(u[2])*cos(u[1])
  (zg.W - zb.B)cY.sX : Fcn  Expr=((zg * W - zb * B) * cos(u[2])) * sin(u[1])
  (zg.W - zb.B)sY : Fcn  Expr=(zg*W - zb*B)*sin(u[2])
  -(xg.W-xb.B)cY.sX : Fcn  Expr=-(xg*W -xb*B)*cos(u[2])*sin(u[1])
  -(yg.W-yb.B)cY.cX : Fcn  Expr=-(yg*W - yb*B)*cos(u[2])*cos(u[1])
  -(yg.W-yb.B)sY : Fcn  Expr=-(yg*W - yb*B)*sin(u[2])
  -cY.cX : Fcn  Expr=-(W-B)*cos(u[2])*cos(u[1])
  -cY.sX : Fcn  Expr=-(W-B)*cos(u[2])*sin(u[1])
  Demux : Demux  Outputs=2
  Mux : Mux  Inputs=3
  Mux1 : Mux
  Sum : Sum  InputSameDT=on  SaturateOnIntegerOverflow=on  OutDataTypeStr=Inherit: Same as first input
  Sum1 : Sum  InputSameDT=on  SaturateOnIntegerOverflow=on  OutDataTypeStr=Inherit: Same as first input
  Sum2 : Sum  InputSameDT=on  SaturateOnIntegerOverflow=on  OutDataTypeStr=Inherit: Same as first input
  Terminator : Terminator
  sY : Fcn  Expr=(W-B)*sin(u[2])
  Gravitational Force : Outport
  wires:
  Demux/1 -> Terminator/1
  Demux/2 -> sY/1, -cY.sX/1, -cY.cX/1, (zg.W - zb.B)cY.sX/1, -(yg.W-yb.B)cY.cX/1, (xg.W-xb.B)cY.cX/1, (zg.W - zb.B)sY/1, -(xg.W-xb.B)cY.sX/1, -(yg.W-yb.B)sY/1
  positions/1 -> Demux/1
  Sum2/1 -> Mux1/4
  sY/1 -> Mux/1
  Mux1/1 -> Gravitational Force/1
  -cY.sX/1 -> Mux/2
  -cY.cX/1 -> Mux/3
  Sum/1 -> Mux1/2
  -(xg.W-xb.B)cY.sX/1 -> Sum2/2
  Sum1/1 -> Mux1/3
  Mux/1 -> Mux1/1
  -(yg.W-yb.B)cY.cX/1 -> Sum/2
  (zg.W - zb.B)cY.sX/1 -> Sum/1
  (xg.W-xb.B)cY.cX/1 -> Sum1/1
  (zg.W - zb.B)sY/1 -> Sum1/2
  -(yg.W-yb.B)sY/1 -> Sum2/1

== system LIVA_AUV_SIMULATOR/6DOF CONTROL/2 DoF i-PID Controller ==
  Earth Frame Reference Trajectory : Inport
  Error Signals : Inport  Port=2
  Earth Frame Positions : Inport  Port=3
  " i-PID Feedback Controller " : Subsystem
  "Feedforward PID Controller " : Subsystem
  Sum : Sum  Inputs=|++
  Control Signals : Outport
  wires:
  Earth Frame Reference Trajectory/1 -> " i-PID Feedback Controller "/1(Body Frame Reference Trajectory), "Feedforward PID Controller "/1(Reference Signals)
  Error Signals/1 -> " i-PID Feedback Controller "/2(Error Signals)
  "Feedforward PID Controller "/1(iPID Control Signals) -> Sum/1
  Earth Frame Positions/1 -> " i-PID Feedback Controller "/3(Body Frame Positions)
  " i-PID Feedback Controller "/1(iPID Control Signals) -> Sum/2
  Sum/1 -> Control Signals/1

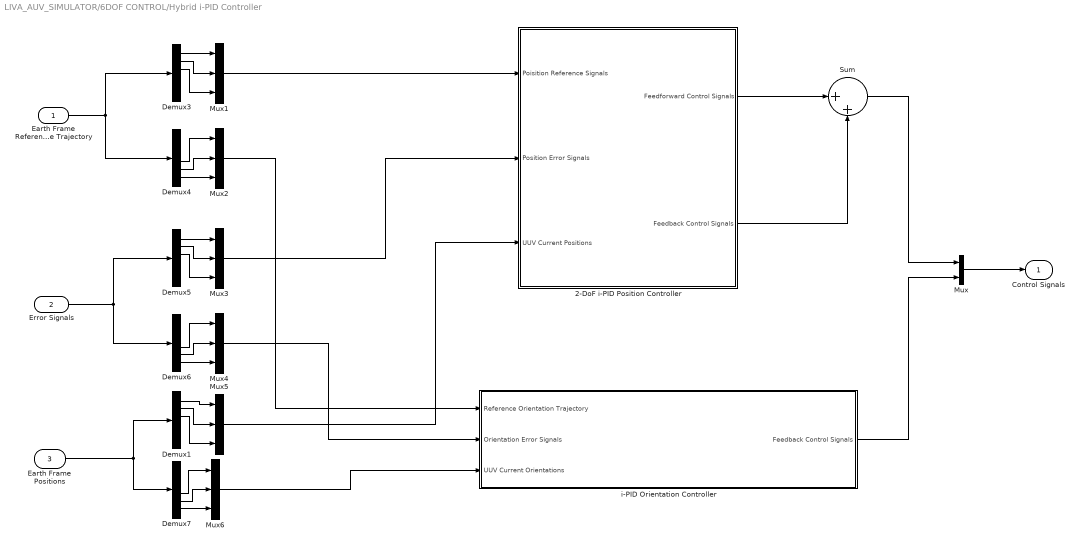
== system LIVA_AUV_SIMULATOR/6DOF CONTROL/Hybrid i-PID Controller ==
  Earth Frame Reference Trajectory : Inport
  Error Signals : Inport  Port=2
  Earth Frame Positions : Inport  Port=3
  2-DoF i-PID Position Controller : Subsystem
  Demux{1,3..7} (6 alike) : Demux  Outputs=6
  Mux : Mux  Inputs=2
  Mux{1..6} (6 alike) : Mux  Inputs=3
  Sum : Sum  Inputs=|++
  i-PID Orientation Controller : Subsystem
  Control Signals : Outport
  wires:
  Mux1/1 -> 2-DoF i-PID Position Controller/1(Poisition Reference Signals)
  Mux3/1 -> 2-DoF i-PID Position Controller/2(Position Error Signals)
  Mux5/1 -> 2-DoF i-PID Position Controller/3(UUV Current Positions)
  2-DoF i-PID Position Controller/1(Feedforward Control Signals) -> Sum/1
  2-DoF i-PID Position Controller/2(Feedback Control Signals) -> Sum/2
  Sum/1 -> Mux/1
  Mux/1 -> Control Signals/1
  i-PID Orientation Controller/1(Feedback Control Signals) -> Mux/2
  Mux2/1 -> i-PID Orientation Controller/1(" Reference Orientation Trajectory")
  Mux4/1 -> i-PID Orientation Controller/2(Orientation Error Signals)
  Mux6/1 -> i-PID Orientation Controller/3(UUV Current Orientations)
  Demux3/1 -> Mux1/1
  Demux3/2 -> Mux1/2
  Demux3/3 -> Mux1/3
  Demux4/4 -> Mux2/1
  Demux4/5 -> Mux2/2
  Demux4/6 -> Mux2/3
  Earth Frame Reference Trajectory/1 -> Demux4/1, Demux3/1
  Demux6/6 -> Mux4/3
  Demux5/3 -> Mux3/3
  Demux5/2 -> Mux3/2
  Demux6/5 -> Mux4/2
  Demux6/4 -> Mux4/1
  Demux5/1 -> Mux3/1
  Error Signals/1 -> Demux5/1, Demux6/1
  Demux7/6 -> Mux6/3
  Demux1/3 -> Mux5/3
  Demux1/2 -> Mux5/2
  Demux7/5 -> Mux6/2
  Demux7/4 -> Mux6/1
  Demux1/1 -> Mux5/1
  Earth Frame Positions/1 -> Demux7/1, Demux1/1
